simulink model "collagenSim"  (R2021b)
settings: Solver=VariableStepAuto  StartTime=0.0  StopTime=900  RelTol=1e-3
libraries: fl_lib x360, nesl_utility x174, rllib x1
(part 2 of 4)

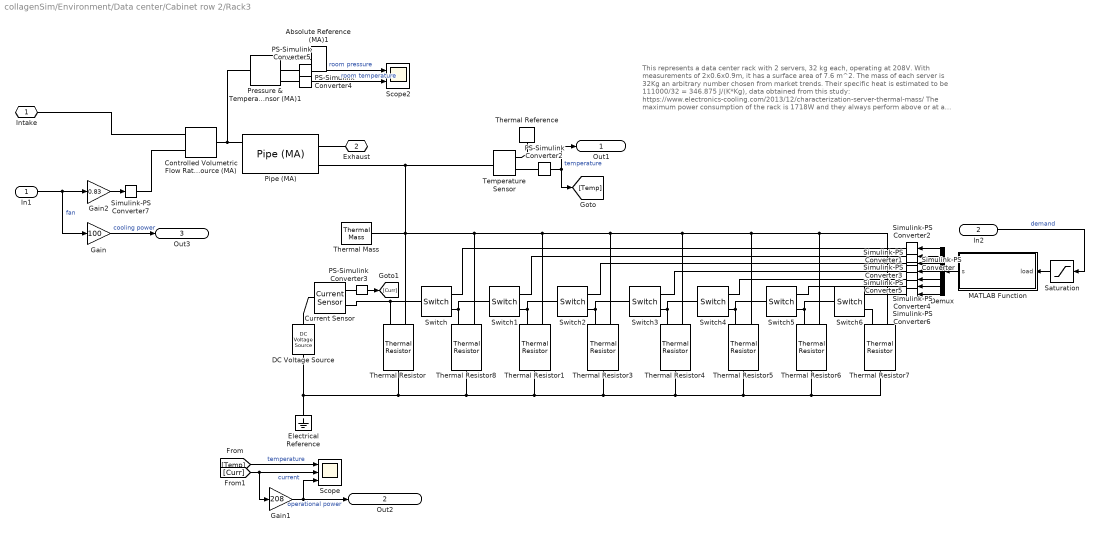
== system collagenSim/Environment/Data center/Cabinet row 2/Rack3 ==
  note: This represents a data center rack with 2 servers, 32 kg each, operating at 208V. With measurements of 2x0.6x0.9m, it has a surface area of 7.6 m^2. The mass of each server is 32Kg an arbitrary number chosen from market trends. Their specific heat is estimated to be 111000/32 = 346.875 J/(K*Kg), data obtained from this study: https://www.electronics-cooling.com/2013/12/characterization-server-thermal-mass/
      | The maximum power consumption of the rack is 1718W and they always perform above or at a minumum of 214.75W.
      | The rack's temperature exchange with the outside environment is modeled with a fluid pipe using the thermal propeties of air at sea level. The cooling system is modeled as eight 8mm four fan panels consuming a maximum of 100W per panel, which gives to each of the eight a total maximum vulumetric rate of 212m^3/min, meaning 0.83m^3/s. The surface area of the pipe representing the interior of the servers has been underestimated to be equal to the surface of the casing that contains them.
  In1 : Inport
  In2 : Inport  Port=2
  Absolute Reference (MA)1 : fl_lib/Moist Air/Elements/Absolute Reference (MA)
      settings: SourceProductBaseCode=SS
  Controlled Volumetric Flow Rate Source (MA) : fl_lib/Moist Air/Sources/Controlled Volumetric Flow Rate Source (MA)  power_spec=foundation.enum.power_spec.isentropic  volumetric_flow_conditions=foundation.enum.volumetric_flow_conditions.actual  p_std=0.101325 MPa  T_std=20 degC  RH_std=0.65  area_A=2*(2*0.442*0.4+2*0.442*0.711) m^2  area_B=2*(2*0.442*0.4+2*0.442*0.711) m^2
      settings: SourceProductBaseCode=SS  InternalSimscapePortConfiguration="{\"Bottom\":[],\"Left\":[{\"id\":\"A\",\"label\":\"A\",\"type\":\"foundation.moist_air.moist_air\"},{\"id\":\"V\",\"label\":\"V\",\"type\":\"input\"}],\"Right\":[{\"id\":\"B\",\"label\":\"B\",\"type\":\"foundation.moist_air.moist_air\"}],\"Top\":[]}"
  Current Sensor : fl_lib/Electrical/Electrical Sensors/Current Sensor
  DC Voltage Source : fl_lib/Electrical/Electrical Sources/DC Voltage Source  v0=208 V
  Demux : Demux  Outputs=7
  Electrical Reference : fl_lib/Electrical/Electrical Elements/Electrical Reference
  Gain : Gain  Gain=100
  Gain1 : Gain  Gain=208
  Gain2 : Gain  Gain=0.83
  MATLAB Function : MATLAB Function  TreatAsAtomicUnit=on
  PS-Simulink Converter{2..5} (4 alike) : nesl_utility/PS-Simulink Converter  PhysicalDomain=network_engine_domain  SubClassName=ps_output  LeftPortType=input  RightPortType=output  PseudoPeriodic=off  Frequencies=[]  Unit=inherit  AffineConversion=off
      settings: SourceProductBaseCode=PW,SS
  Pipe (MA) : fl_lib/Moist Air/Elements/Pipe (MA)  length=0.711 m  area=2*(2*0.442*0.4+2*0.442*0.711) m^2  Dh=0.1 m  length_add=0.1 m  roughness=15e-6 m  Re_lam=2000  Re_tur=4000  shape_factor=64  Nu_lam=3.66  RH_ws=1  time_constant=1e-3 s  moisture_trace_gas_source=foundation.enum.moisture_trace_gas_source.none  moisture_source_spec=foundation.enum.moisture_source_spec.vapor  moisture_mass_flow=0 kg/s  moisture_temperature_spec=foundation.enum.temperature_spec.atmospheric  moisture_temperature=293.15 K  trace_gas_mass_flow=0 kg/s  trace_gas_temperature_spec=foundation.enum.temperature_spec.atmospheric  trace_gas_temperature=293.15 K  p_I_specify=off  p_I_priority=High  p_I=0.101325 MPa  p_I_nominal_specify=off  p_I_nominal_unit=MPa  p_I_nominal_value=1  T_I_specify=off  T_I_priority=High  T_I=293.15 K  T_I_nominal_specify=off  T_I_nominal_unit=K  T_I_nominal_value=1  RH_I_specify=off  RH_I_priority=High  RH_I=0  RH_I_nominal_specify=off  RH_I_nominal_unit=1  RH_I_nominal_value=1  x_w_I_specify=off  x_w_I_priority=None  x_w_I=0  x_w_I_nominal_specify=off  x_w_I_nominal_unit=1  x_w_I_nominal_value=1  y_w_I_specify=off  y_w_I_priority=None  y_w_I=0  y_w_I_nominal_specify=off  y_w_I_nominal_unit=1  y_w_I_nominal_value=1  HR_I_specify=off  HR_I_priority=None  HR_I=0  HR_I_nominal_specify=off  HR_I_nominal_unit=1  HR_I_nominal_value=1  x_g_I_specify=off  x_g_I_priority=High  x_g_I=0  x_g_I_nominal_specify=off  x_g_I_nominal_unit=1  x_g_I_nominal_value=1  y_g_I_specify=off  y_g_I_priority=None  y_g_I=0  y_g_I_nominal_specify=off  y_g_I_nominal_unit=1  y_g_I_nominal_value=1
      settings: SourceProductBaseCode=SS
  Pressure & Temperature Sensor (MA)1 : fl_lib/Moist Air/Sensors/Pressure & Temperature Sensor (MA)
      settings: SourceProductBaseCode=SS  InternalSimscapePortConfiguration="{\"Bottom\":[],\"Left\":[{\"id\":\"A\",\"label\":\"A\",\"type\":\"foundation.moist_air.moist_air\"}],\"Right\":[{\"id\":\"B\",\"label\":\"B\",\"type\":\"foundation.moist_air.moist_air\"},{\"id\":\"P\",\"label\":\"P\",\"type\":\"output\"},{\"id\":\"T\",\"label\":\"T\",\"type\":\"output\"}],\"Top\":[]}"
  Saturation : Saturate  UpperLimit=0.99  LowerLimit=0.01
  Scope : Scope  NumInputPorts=3
  Scope2 : Scope  NumInputPorts=2
  Simulink-PS Converter{,1..7} (8 alike) : nesl_utility/Simulink-PS Converter  PhysicalDomain=network_engine_domain  SubClassName=ps_input  LeftPortType=input  RightPortType=output  PseudoPeriodic=off  Frequencies=[]  NoiseDistribution=none  NoiseParameters=[]  Unit=1  AffineConversion=off  FilteringAndDerivatives=provide  SimscapeFilterOrder=1  InputFilterTimeConstant=0.001  UdotUserProvided=0
      settings: SourceProductBaseCode=PW,SS
  Switch{,1..6} (7 alike) : fl_lib/Electrical/Electrical Elements/Switch  R_closed=0.01 Ohm  G_open=1e-8 1/Ohm  Threshold=0.5  i_specify=off  i_priority=None  i=0 A  i_nominal_specify=off  i_nominal_unit=A  i_nominal_value=1  v_specify=off  v_priority=None  v=0 V  v_nominal_specify=off  v_nominal_unit=V  v_nominal_value=1
  Temperature Sensor : fl_lib/Thermal/Thermal Sensors/Temperature Sensor
  Thermal Mass : fl_lib/Thermal/Thermal Elements/Thermal Mass  mass=64 kg  sp_heat=346.875 J/(K*kg)  T_specify=on  T_priority=High  T=293.15 K  T_nominal_specify=off  T_nominal_unit=K  T_nominal_value=1  Q_specify=off  Q_priority=None  Q=0 W  Q_nominal_specify=off  Q_nominal_unit=W  Q_nominal_value=1
  Thermal Reference : fl_lib/Thermal/Thermal Elements/Thermal Reference
  Thermal Resistor{,1,3..8} (8 alike) : fl_lib/Electrical/Electrical Elements/Thermal Resistor  R0=208^2/1718*8 Ohm  T0=298.15 K  alpha=50e-6 1/K  tc=10 s  K_d=1e-3 W/K  T_specify=on  T_priority=High  T=293.15 K  T_nominal_specify=off  T_nominal_unit=K  T_nominal_value=1
      settings: SourceProductBaseCode=SS  InternalSimscapePortConfiguration="{\"Bottom\":[],\"Left\":[{\"id\":\"H\",\"label\":\"H\",\"type\":\"foundation.thermal.thermal\"},{\"id\":\"p\",\"label\":\"+\",\"type\":\"foundation.electrical.electrical\"}],\"Right\":[{\"id\":\"n\",\"label\":\"-\",\"type\":\"foundation.electrical.electrical\"}],\"Top\":[]}"
  Intake : PMIOPort  Side=Left
  Exhaust : PMIOPort  Port=2  Side=Right
  Out1 : Outport
  Out2 : Outport  Port=2
  Out3 : Outport  Port=3
  wires:
  Demux/6 -> Simulink-PS Converter5/1
  Demux/1 -> Simulink-PS Converter2/1
  Demux/2 -> Simulink-PS Converter1/1
  Demux/7 -> Simulink-PS Converter6/1
  PS-Simulink Converter2/1 -> Out1/1, [Temp]  "temperature"
  [Curr] -> Scope/2, Gain1/1  "current"
  [Temp] -> Scope/1  "temperature"
  PS-Simulink Converter3/1 -> [Curr]
  Saturation/1 -> MATLAB Function/1(load)
  In2/1 -> Saturation/1  "demand"
  Demux/4 -> Simulink-PS Converter3/1
  Demux/3 -> Simulink-PS Converter/1
  Demux/5 -> Simulink-PS Converter4/1
  MATLAB Function/1(s) -> Demux/1
  Gain1/1 -> Out2/1, Scope/3  "operational power"
  In1/1 -> Gain/1, Gain2/1  "fan"
  Gain2/1 -> Simulink-PS Converter7/1
  Gain/1 -> Out3/1  "cooling power"
  PS-Simulink Converter5/1 -> Scope2/1  "room pressure"
  PS-Simulink Converter4/1 -> Scope2/2  "room temperature"
  connections:
  Switch3/LConn1 -- Switch2/RConn2 -- Thermal Resistor3/LConn2
  Thermal Resistor3/RConn1 -- Thermal Resistor6/RConn1 -- Thermal Resistor7/RConn1 -- Thermal Resistor5/RConn1 -- Thermal Resistor4/RConn1 -- Thermal Resistor8/RConn1 -- Electrical Reference/LConn1 -- DC Voltage Source/RConn1 -- Thermal Resistor/RConn1 -- Thermal Resistor1/RConn1
  DC Voltage Source/LConn1 -- Current Sensor/LConn1
  Switch2/LConn1 -- Switch1/RConn2 -- Thermal Resistor1/LConn2
  Switch1/LConn1 -- Switch/RConn2 -- Thermal Resistor8/LConn2
  Thermal Resistor4/LConn2 -- Switch4/LConn1 -- Switch3/RConn2
  Switch6/LConn1 -- Switch5/RConn2 -- Thermal Resistor6/LConn2
  Switch/LConn1 -- Current Sensor/RConn2 -- Thermal Resistor/LConn2
  Thermal Resistor5/LConn2 -- Switch5/LConn1 -- Switch4/RConn2
  Thermal Reference/LConn1 -- Temperature Sensor/RConn1
  Simulink-PS Converter6/RConn1 -- Switch6/RConn1
  Thermal Resistor7/LConn2 -- Switch6/RConn2
  Simulink-PS Converter4/RConn1 -- Switch4/RConn1
  Simulink-PS Converter2/RConn1 -- Switch/RConn1
  Simulink-PS Converter1/RConn1 -- Switch1/RConn1
  Temperature Sensor/RConn2 -- PS-Simulink Converter2/LConn1
  Simulink-PS Converter/RConn1 -- Switch2/RConn1
  Current Sensor/RConn1 -- PS-Simulink Converter3/LConn1
  Simulink-PS Converter3/RConn1 -- Switch3/RConn1
  Simulink-PS Converter5/RConn1 -- Switch5/RConn1
  Controlled Volumetric Flow Rate Source (MA)/LConn2 -- Simulink-PS Converter7/RConn1
  Pipe (MA)/RConn1 -- Controlled Volumetric Flow Rate Source (MA)/RConn1 -- Pressure & Temperature Sensor (MA)1/LConn1
  Intake/RConn1 -- Controlled Volumetric Flow Rate Source (MA)/LConn1
  Pipe (MA)/LConn1 -- Exhaust/RConn1
  Thermal Resistor8/LConn1 -- Pipe (MA)/LConn2 -- Temperature Sensor/LConn1 -- Thermal Resistor/LConn1 -- Thermal Mass/LConn1 -- Thermal Resistor6/LConn1 -- Thermal Resistor7/LConn1 -- Thermal Resistor5/LConn1 -- Thermal Resistor4/LConn1 -- Thermal Resistor3/LConn1 -- Thermal Resistor1/LConn1
  PS-Simulink Converter5/LConn1 -- Pressure & Temperature Sensor (MA)1/RConn2
  PS-Simulink Converter4/LConn1 -- Pressure & Temperature Sensor (MA)1/RConn3
  Absolute Reference (MA)1/LConn1 -- Pressure & Temperature Sensor (MA)1/RConn1

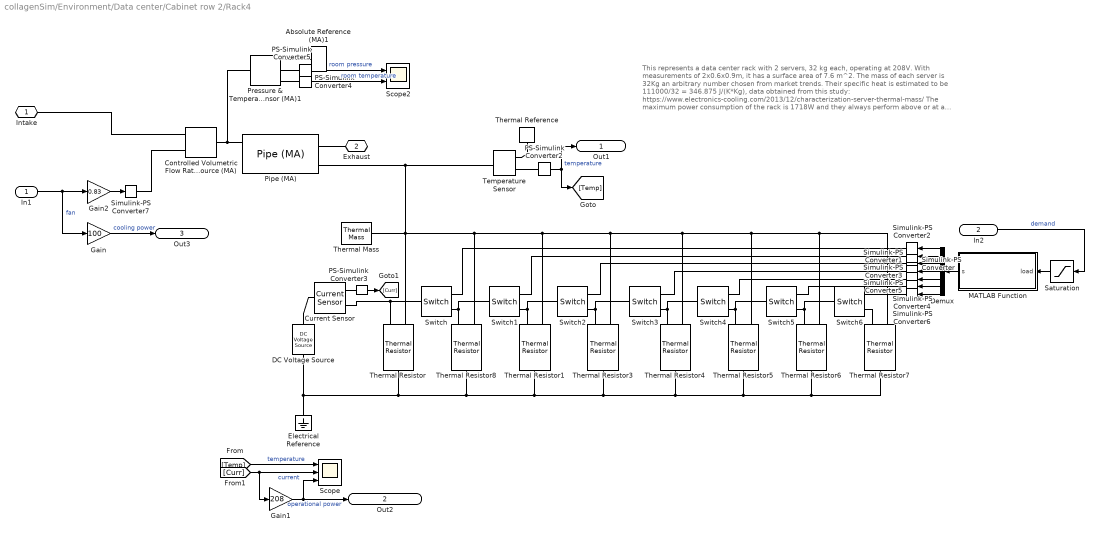
== system collagenSim/Environment/Data center/Cabinet row 2/Rack4 ==
  note: This represents a data center rack with 2 servers, 32 kg each, operating at 208V. With measurements of 2x0.6x0.9m, it has a surface area of 7.6 m^2. The mass of each server is 32Kg an arbitrary number chosen from market trends. Their specific heat is estimated to be 111000/32 = 346.875 J/(K*Kg), data obtained from this study: https://www.electronics-cooling.com/2013/12/characterization-server-thermal-mass/
      | The maximum power consumption of the rack is 1718W and they always perform above or at a minumum of 214.75W.
      | The rack's temperature exchange with the outside environment is modeled with a fluid pipe using the thermal propeties of air at sea level. The cooling system is modeled as eight 8mm four fan panels consuming a maximum of 100W per panel, which gives to each of the eight a total maximum vulumetric rate of 212m^3/min, meaning 0.83m^3/s. The surface area of the pipe representing the interior of the servers has been underestimated to be equal to the surface of the casing that contains them.
  In1 : Inport
  In2 : Inport  Port=2
  Absolute Reference (MA)1 : fl_lib/Moist Air/Elements/Absolute Reference (MA)
      settings: SourceProductBaseCode=SS
  Controlled Volumetric Flow Rate Source (MA) : fl_lib/Moist Air/Sources/Controlled Volumetric Flow Rate Source (MA)  power_spec=foundation.enum.power_spec.isentropic  volumetric_flow_conditions=foundation.enum.volumetric_flow_conditions.actual  p_std=0.101325 MPa  T_std=20 degC  RH_std=0.65  area_A=2*(2*0.442*0.4+2*0.442*0.711) m^2  area_B=2*(2*0.442*0.4+2*0.442*0.711) m^2
      settings: SourceProductBaseCode=SS  InternalSimscapePortConfiguration="{\"Bottom\":[],\"Left\":[{\"id\":\"A\",\"label\":\"A\",\"type\":\"foundation.moist_air.moist_air\"},{\"id\":\"V\",\"label\":\"V\",\"type\":\"input\"}],\"Right\":[{\"id\":\"B\",\"label\":\"B\",\"type\":\"foundation.moist_air.moist_air\"}],\"Top\":[]}"
  Current Sensor : fl_lib/Electrical/Electrical Sensors/Current Sensor
  DC Voltage Source : fl_lib/Electrical/Electrical Sources/DC Voltage Source  v0=208 V
  Demux : Demux  Outputs=7
  Electrical Reference : fl_lib/Electrical/Electrical Elements/Electrical Reference
  Gain : Gain  Gain=100
  Gain1 : Gain  Gain=208
  Gain2 : Gain  Gain=0.83
  MATLAB Function : MATLAB Function  TreatAsAtomicUnit=on
  PS-Simulink Converter{2..5} (4 alike) : nesl_utility/PS-Simulink Converter  PhysicalDomain=network_engine_domain  SubClassName=ps_output  LeftPortType=input  RightPortType=output  PseudoPeriodic=off  Frequencies=[]  Unit=inherit  AffineConversion=off
      settings: SourceProductBaseCode=PW,SS
  Pipe (MA) : fl_lib/Moist Air/Elements/Pipe (MA)  length=0.711 m  area=2*(2*0.442*0.4+2*0.442*0.711) m^2  Dh=0.1 m  length_add=0.1 m  roughness=15e-6 m  Re_lam=2000  Re_tur=4000  shape_factor=64  Nu_lam=3.66  RH_ws=1  time_constant=1e-3 s  moisture_trace_gas_source=foundation.enum.moisture_trace_gas_source.none  moisture_source_spec=foundation.enum.moisture_source_spec.vapor  moisture_mass_flow=0 kg/s  moisture_temperature_spec=foundation.enum.temperature_spec.atmospheric  moisture_temperature=293.15 K  trace_gas_mass_flow=0 kg/s  trace_gas_temperature_spec=foundation.enum.temperature_spec.atmospheric  trace_gas_temperature=293.15 K  p_I_specify=off  p_I_priority=High  p_I=0.101325 MPa  p_I_nominal_specify=off  p_I_nominal_unit=MPa  p_I_nominal_value=1  T_I_specify=off  T_I_priority=High  T_I=293.15 K  T_I_nominal_specify=off  T_I_nominal_unit=K  T_I_nominal_value=1  RH_I_specify=off  RH_I_priority=High  RH_I=0  RH_I_nominal_specify=off  RH_I_nominal_unit=1  RH_I_nominal_value=1  x_w_I_specify=off  x_w_I_priority=None  x_w_I=0  x_w_I_nominal_specify=off  x_w_I_nominal_unit=1  x_w_I_nominal_value=1  y_w_I_specify=off  y_w_I_priority=None  y_w_I=0  y_w_I_nominal_specify=off  y_w_I_nominal_unit=1  y_w_I_nominal_value=1  HR_I_specify=off  HR_I_priority=None  HR_I=0  HR_I_nominal_specify=off  HR_I_nominal_unit=1  HR_I_nominal_value=1  x_g_I_specify=off  x_g_I_priority=High  x_g_I=0  x_g_I_nominal_specify=off  x_g_I_nominal_unit=1  x_g_I_nominal_value=1  y_g_I_specify=off  y_g_I_priority=None  y_g_I=0  y_g_I_nominal_specify=off  y_g_I_nominal_unit=1  y_g_I_nominal_value=1
      settings: SourceProductBaseCode=SS
  Pressure & Temperature Sensor (MA)1 : fl_lib/Moist Air/Sensors/Pressure & Temperature Sensor (MA)
      settings: SourceProductBaseCode=SS  InternalSimscapePortConfiguration="{\"Bottom\":[],\"Left\":[{\"id\":\"A\",\"label\":\"A\",\"type\":\"foundation.moist_air.moist_air\"}],\"Right\":[{\"id\":\"B\",\"label\":\"B\",\"type\":\"foundation.moist_air.moist_air\"},{\"id\":\"P\",\"label\":\"P\",\"type\":\"output\"},{\"id\":\"T\",\"label\":\"T\",\"type\":\"output\"}],\"Top\":[]}"
  Saturation : Saturate  UpperLimit=0.99  LowerLimit=0.01
  Scope : Scope  NumInputPorts=3
  Scope2 : Scope  NumInputPorts=2
  Simulink-PS Converter{,1..7} (8 alike) : nesl_utility/Simulink-PS Converter  PhysicalDomain=network_engine_domain  SubClassName=ps_input  LeftPortType=input  RightPortType=output  PseudoPeriodic=off  Frequencies=[]  NoiseDistribution=none  NoiseParameters=[]  Unit=1  AffineConversion=off  FilteringAndDerivatives=provide  SimscapeFilterOrder=1  InputFilterTimeConstant=0.001  UdotUserProvided=0
      settings: SourceProductBaseCode=PW,SS
  Switch{,1..6} (7 alike) : fl_lib/Electrical/Electrical Elements/Switch  R_closed=0.01 Ohm  G_open=1e-8 1/Ohm  Threshold=0.5  i_specify=off  i_priority=None  i=0 A  i_nominal_specify=off  i_nominal_unit=A  i_nominal_value=1  v_specify=off  v_priority=None  v=0 V  v_nominal_specify=off  v_nominal_unit=V  v_nominal_value=1
  Temperature Sensor : fl_lib/Thermal/Thermal Sensors/Temperature Sensor
  Thermal Mass : fl_lib/Thermal/Thermal Elements/Thermal Mass  mass=64 kg  sp_heat=346.875 J/(K*kg)  T_specify=on  T_priority=High  T=293.15 K  T_nominal_specify=off  T_nominal_unit=K  T_nominal_value=1  Q_specify=off  Q_priority=None  Q=0 W  Q_nominal_specify=off  Q_nominal_unit=W  Q_nominal_value=1
  Thermal Reference : fl_lib/Thermal/Thermal Elements/Thermal Reference
  Thermal Resistor{,1,3..8} (8 alike) : fl_lib/Electrical/Electrical Elements/Thermal Resistor  R0=208^2/1718*8 Ohm  T0=298.15 K  alpha=50e-6 1/K  tc=10 s  K_d=1e-3 W/K  T_specify=on  T_priority=High  T=293.15 K  T_nominal_specify=off  T_nominal_unit=K  T_nominal_value=1
      settings: SourceProductBaseCode=SS  InternalSimscapePortConfiguration="{\"Bottom\":[],\"Left\":[{\"id\":\"H\",\"label\":\"H\",\"type\":\"foundation.thermal.thermal\"},{\"id\":\"p\",\"label\":\"+\",\"type\":\"foundation.electrical.electrical\"}],\"Right\":[{\"id\":\"n\",\"label\":\"-\",\"type\":\"foundation.electrical.electrical\"}],\"Top\":[]}"
  Intake : PMIOPort  Side=Left
  Exhaust : PMIOPort  Port=2  Side=Right
  Out1 : Outport
  Out2 : Outport  Port=2
  Out3 : Outport  Port=3
  wires:
  Demux/6 -> Simulink-PS Converter5/1
  Demux/1 -> Simulink-PS Converter2/1
  Demux/2 -> Simulink-PS Converter1/1
  Demux/7 -> Simulink-PS Converter6/1
  PS-Simulink Converter2/1 -> Out1/1, [Temp]  "temperature"
  [Curr] -> Scope/2, Gain1/1  "current"
  [Temp] -> Scope/1  "temperature"
  PS-Simulink Converter3/1 -> [Curr]
  Saturation/1 -> MATLAB Function/1(load)
  In2/1 -> Saturation/1  "demand"
  Demux/4 -> Simulink-PS Converter3/1
  Demux/3 -> Simulink-PS Converter/1
  Demux/5 -> Simulink-PS Converter4/1
  MATLAB Function/1(s) -> Demux/1
  Gain1/1 -> Out2/1, Scope/3  "operational power"
  In1/1 -> Gain/1, Gain2/1  "fan"
  Gain2/1 -> Simulink-PS Converter7/1
  Gain/1 -> Out3/1  "cooling power"
  PS-Simulink Converter5/1 -> Scope2/1  "room pressure"
  PS-Simulink Converter4/1 -> Scope2/2  "room temperature"
  connections:
  Switch3/LConn1 -- Switch2/RConn2 -- Thermal Resistor3/LConn2
  Thermal Resistor3/RConn1 -- Thermal Resistor6/RConn1 -- Thermal Resistor7/RConn1 -- Thermal Resistor5/RConn1 -- Thermal Resistor4/RConn1 -- Thermal Resistor8/RConn1 -- Electrical Reference/LConn1 -- DC Voltage Source/RConn1 -- Thermal Resistor/RConn1 -- Thermal Resistor1/RConn1
  DC Voltage Source/LConn1 -- Current Sensor/LConn1
  Switch2/LConn1 -- Switch1/RConn2 -- Thermal Resistor1/LConn2
  Switch1/LConn1 -- Switch/RConn2 -- Thermal Resistor8/LConn2
  Thermal Resistor4/LConn2 -- Switch4/LConn1 -- Switch3/RConn2
  Switch6/LConn1 -- Switch5/RConn2 -- Thermal Resistor6/LConn2
  Switch/LConn1 -- Current Sensor/RConn2 -- Thermal Resistor/LConn2
  Thermal Resistor5/LConn2 -- Switch5/LConn1 -- Switch4/RConn2
  Thermal Reference/LConn1 -- Temperature Sensor/RConn1
  Simulink-PS Converter6/RConn1 -- Switch6/RConn1
  Thermal Resistor7/LConn2 -- Switch6/RConn2
  Simulink-PS Converter4/RConn1 -- Switch4/RConn1
  Simulink-PS Converter2/RConn1 -- Switch/RConn1
  Simulink-PS Converter1/RConn1 -- Switch1/RConn1
  Temperature Sensor/RConn2 -- PS-Simulink Converter2/LConn1
  Simulink-PS Converter/RConn1 -- Switch2/RConn1
  Current Sensor/RConn1 -- PS-Simulink Converter3/LConn1
  Simulink-PS Converter3/RConn1 -- Switch3/RConn1
  Simulink-PS Converter5/RConn1 -- Switch5/RConn1
  Controlled Volumetric Flow Rate Source (MA)/LConn2 -- Simulink-PS Converter7/RConn1
  Pipe (MA)/RConn1 -- Controlled Volumetric Flow Rate Source (MA)/RConn1 -- Pressure & Temperature Sensor (MA)1/LConn1
  Intake/RConn1 -- Controlled Volumetric Flow Rate Source (MA)/LConn1
  Pipe (MA)/LConn1 -- Exhaust/RConn1
  Thermal Resistor8/LConn1 -- Pipe (MA)/LConn2 -- Temperature Sensor/LConn1 -- Thermal Resistor/LConn1 -- Thermal Mass/LConn1 -- Thermal Resistor6/LConn1 -- Thermal Resistor7/LConn1 -- Thermal Resistor5/LConn1 -- Thermal Resistor4/LConn1 -- Thermal Resistor3/LConn1 -- Thermal Resistor1/LConn1
  PS-Simulink Converter5/LConn1 -- Pressure & Temperature Sensor (MA)1/RConn2
  PS-Simulink Converter4/LConn1 -- Pressure & Temperature Sensor (MA)1/RConn3
  Absolute Reference (MA)1/LConn1 -- Pressure & Temperature Sensor (MA)1/RConn1

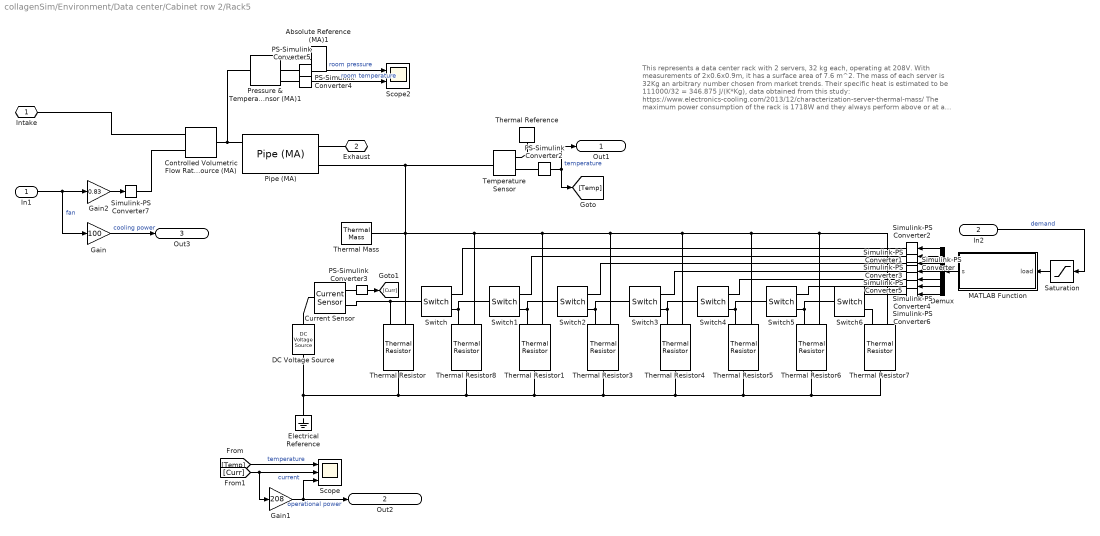
== system collagenSim/Environment/Data center/Cabinet row 2/Rack5 ==
  note: This represents a data center rack with 2 servers, 32 kg each, operating at 208V. With measurements of 2x0.6x0.9m, it has a surface area of 7.6 m^2. The mass of each server is 32Kg an arbitrary number chosen from market trends. Their specific heat is estimated to be 111000/32 = 346.875 J/(K*Kg), data obtained from this study: https://www.electronics-cooling.com/2013/12/characterization-server-thermal-mass/
      | The maximum power consumption of the rack is 1718W and they always perform above or at a minumum of 214.75W.
      | The rack's temperature exchange with the outside environment is modeled with a fluid pipe using the thermal propeties of air at sea level. The cooling system is modeled as eight 8mm four fan panels consuming a maximum of 100W per panel, which gives to each of the eight a total maximum vulumetric rate of 212m^3/min, meaning 0.83m^3/s. The surface area of the pipe representing the interior of the servers has been underestimated to be equal to the surface of the casing that contains them.
  In1 : Inport
  In2 : Inport  Port=2
  Absolute Reference (MA)1 : fl_lib/Moist Air/Elements/Absolute Reference (MA)
      settings: SourceProductBaseCode=SS
  Controlled Volumetric Flow Rate Source (MA) : fl_lib/Moist Air/Sources/Controlled Volumetric Flow Rate Source (MA)  power_spec=foundation.enum.power_spec.isentropic  volumetric_flow_conditions=foundation.enum.volumetric_flow_conditions.actual  p_std=0.101325 MPa  T_std=20 degC  RH_std=0.65  area_A=2*(2*0.442*0.4+2*0.442*0.711) m^2  area_B=2*(2*0.442*0.4+2*0.442*0.711) m^2
      settings: SourceProductBaseCode=SS  InternalSimscapePortConfiguration="{\"Bottom\":[],\"Left\":[{\"id\":\"A\",\"label\":\"A\",\"type\":\"foundation.moist_air.moist_air\"},{\"id\":\"V\",\"label\":\"V\",\"type\":\"input\"}],\"Right\":[{\"id\":\"B\",\"label\":\"B\",\"type\":\"foundation.moist_air.moist_air\"}],\"Top\":[]}"
  Current Sensor : fl_lib/Electrical/Electrical Sensors/Current Sensor
  DC Voltage Source : fl_lib/Electrical/Electrical Sources/DC Voltage Source  v0=208 V
  Demux : Demux  Outputs=7
  Electrical Reference : fl_lib/Electrical/Electrical Elements/Electrical Reference
  Gain : Gain  Gain=100
  Gain1 : Gain  Gain=208
  Gain2 : Gain  Gain=0.83
  MATLAB Function : MATLAB Function  TreatAsAtomicUnit=on
  PS-Simulink Converter{2..5} (4 alike) : nesl_utility/PS-Simulink Converter  PhysicalDomain=network_engine_domain  SubClassName=ps_output  LeftPortType=input  RightPortType=output  PseudoPeriodic=off  Frequencies=[]  Unit=inherit  AffineConversion=off
      settings: SourceProductBaseCode=PW,SS
  Pipe (MA) : fl_lib/Moist Air/Elements/Pipe (MA)  length=0.711 m  area=2*(2*0.442*0.4+2*0.442*0.711) m^2  Dh=0.1 m  length_add=0.1 m  roughness=15e-6 m  Re_lam=2000  Re_tur=4000  shape_factor=64  Nu_lam=3.66  RH_ws=1  time_constant=1e-3 s  moisture_trace_gas_source=foundation.enum.moisture_trace_gas_source.none  moisture_source_spec=foundation.enum.moisture_source_spec.vapor  moisture_mass_flow=0 kg/s  moisture_temperature_spec=foundation.enum.temperature_spec.atmospheric  moisture_temperature=293.15 K  trace_gas_mass_flow=0 kg/s  trace_gas_temperature_spec=foundation.enum.temperature_spec.atmospheric  trace_gas_temperature=293.15 K  p_I_specify=off  p_I_priority=High  p_I=0.101325 MPa  p_I_nominal_specify=off  p_I_nominal_unit=MPa  p_I_nominal_value=1  T_I_specify=off  T_I_priority=High  T_I=293.15 K  T_I_nominal_specify=off  T_I_nominal_unit=K  T_I_nominal_value=1  RH_I_specify=off  RH_I_priority=High  RH_I=0  RH_I_nominal_specify=off  RH_I_nominal_unit=1  RH_I_nominal_value=1  x_w_I_specify=off  x_w_I_priority=None  x_w_I=0  x_w_I_nominal_specify=off  x_w_I_nominal_unit=1  x_w_I_nominal_value=1  y_w_I_specify=off  y_w_I_priority=None  y_w_I=0  y_w_I_nominal_specify=off  y_w_I_nominal_unit=1  y_w_I_nominal_value=1  HR_I_specify=off  HR_I_priority=None  HR_I=0  HR_I_nominal_specify=off  HR_I_nominal_unit=1  HR_I_nominal_value=1  x_g_I_specify=off  x_g_I_priority=High  x_g_I=0  x_g_I_nominal_specify=off  x_g_I_nominal_unit=1  x_g_I_nominal_value=1  y_g_I_specify=off  y_g_I_priority=None  y_g_I=0  y_g_I_nominal_specify=off  y_g_I_nominal_unit=1  y_g_I_nominal_value=1
      settings: SourceProductBaseCode=SS
  Pressure & Temperature Sensor (MA)1 : fl_lib/Moist Air/Sensors/Pressure & Temperature Sensor (MA)
      settings: SourceProductBaseCode=SS  InternalSimscapePortConfiguration="{\"Bottom\":[],\"Left\":[{\"id\":\"A\",\"label\":\"A\",\"type\":\"foundation.moist_air.moist_air\"}],\"Right\":[{\"id\":\"B\",\"label\":\"B\",\"type\":\"foundation.moist_air.moist_air\"},{\"id\":\"P\",\"label\":\"P\",\"type\":\"output\"},{\"id\":\"T\",\"label\":\"T\",\"type\":\"output\"}],\"Top\":[]}"
  Saturation : Saturate  UpperLimit=0.99  LowerLimit=0.01
  Scope : Scope  NumInputPorts=3
  Scope2 : Scope  NumInputPorts=2
  Simulink-PS Converter{,1..7} (8 alike) : nesl_utility/Simulink-PS Converter  PhysicalDomain=network_engine_domain  SubClassName=ps_input  LeftPortType=input  RightPortType=output  PseudoPeriodic=off  Frequencies=[]  NoiseDistribution=none  NoiseParameters=[]  Unit=1  AffineConversion=off  FilteringAndDerivatives=provide  SimscapeFilterOrder=1  InputFilterTimeConstant=0.001  UdotUserProvided=0
      settings: SourceProductBaseCode=PW,SS
  Switch{,1..6} (7 alike) : fl_lib/Electrical/Electrical Elements/Switch  R_closed=0.01 Ohm  G_open=1e-8 1/Ohm  Threshold=0.5  i_specify=off  i_priority=None  i=0 A  i_nominal_specify=off  i_nominal_unit=A  i_nominal_value=1  v_specify=off  v_priority=None  v=0 V  v_nominal_specify=off  v_nominal_unit=V  v_nominal_value=1
  Temperature Sensor : fl_lib/Thermal/Thermal Sensors/Temperature Sensor
  Thermal Mass : fl_lib/Thermal/Thermal Elements/Thermal Mass  mass=64 kg  sp_heat=346.875 J/(K*kg)  T_specify=on  T_priority=High  T=293.15 K  T_nominal_specify=off  T_nominal_unit=K  T_nominal_value=1  Q_specify=off  Q_priority=None  Q=0 W  Q_nominal_specify=off  Q_nominal_unit=W  Q_nominal_value=1
  Thermal Reference : fl_lib/Thermal/Thermal Elements/Thermal Reference
  Thermal Resistor{,1,3..8} (8 alike) : fl_lib/Electrical/Electrical Elements/Thermal Resistor  R0=208^2/1718*8 Ohm  T0=298.15 K  alpha=50e-6 1/K  tc=10 s  K_d=1e-3 W/K  T_specify=on  T_priority=High  T=293.15 K  T_nominal_specify=off  T_nominal_unit=K  T_nominal_value=1
      settings: SourceProductBaseCode=SS  InternalSimscapePortConfiguration="{\"Bottom\":[],\"Left\":[{\"id\":\"H\",\"label\":\"H\",\"type\":\"foundation.thermal.thermal\"},{\"id\":\"p\",\"label\":\"+\",\"type\":\"foundation.electrical.electrical\"}],\"Right\":[{\"id\":\"n\",\"label\":\"-\",\"type\":\"foundation.electrical.electrical\"}],\"Top\":[]}"
  Intake : PMIOPort  Side=Left
  Exhaust : PMIOPort  Port=2  Side=Right
  Out1 : Outport
  Out2 : Outport  Port=2
  Out3 : Outport  Port=3
  wires:
  Demux/6 -> Simulink-PS Converter5/1
  Demux/1 -> Simulink-PS Converter2/1
  Demux/2 -> Simulink-PS Converter1/1
  Demux/7 -> Simulink-PS Converter6/1
  PS-Simulink Converter2/1 -> Out1/1, [Temp]  "temperature"
  [Curr] -> Scope/2, Gain1/1  "current"
  [Temp] -> Scope/1  "temperature"
  PS-Simulink Converter3/1 -> [Curr]
  Saturation/1 -> MATLAB Function/1(load)
  In2/1 -> Saturation/1  "demand"
  Demux/4 -> Simulink-PS Converter3/1
  Demux/3 -> Simulink-PS Converter/1
  Demux/5 -> Simulink-PS Converter4/1
  MATLAB Function/1(s) -> Demux/1
  Gain1/1 -> Out2/1, Scope/3  "operational power"
  In1/1 -> Gain/1, Gain2/1  "fan"
  Gain2/1 -> Simulink-PS Converter7/1
  Gain/1 -> Out3/1  "cooling power"
  PS-Simulink Converter5/1 -> Scope2/1  "room pressure"
  PS-Simulink Converter4/1 -> Scope2/2  "room temperature"
  connections:
  Switch3/LConn1 -- Switch2/RConn2 -- Thermal Resistor3/LConn2
  Thermal Resistor3/RConn1 -- Thermal Resistor6/RConn1 -- Thermal Resistor7/RConn1 -- Thermal Resistor5/RConn1 -- Thermal Resistor4/RConn1 -- Thermal Resistor8/RConn1 -- Electrical Reference/LConn1 -- DC Voltage Source/RConn1 -- Thermal Resistor/RConn1 -- Thermal Resistor1/RConn1
  DC Voltage Source/LConn1 -- Current Sensor/LConn1
  Switch2/LConn1 -- Switch1/RConn2 -- Thermal Resistor1/LConn2
  Switch1/LConn1 -- Switch/RConn2 -- Thermal Resistor8/LConn2
  Thermal Resistor4/LConn2 -- Switch4/LConn1 -- Switch3/RConn2
  Switch6/LConn1 -- Switch5/RConn2 -- Thermal Resistor6/LConn2
  Switch/LConn1 -- Current Sensor/RConn2 -- Thermal Resistor/LConn2
  Thermal Resistor5/LConn2 -- Switch5/LConn1 -- Switch4/RConn2
  Thermal Reference/LConn1 -- Temperature Sensor/RConn1
  Simulink-PS Converter6/RConn1 -- Switch6/RConn1
  Thermal Resistor7/LConn2 -- Switch6/RConn2
  Simulink-PS Converter4/RConn1 -- Switch4/RConn1
  Simulink-PS Converter2/RConn1 -- Switch/RConn1
  Simulink-PS Converter1/RConn1 -- Switch1/RConn1
  Temperature Sensor/RConn2 -- PS-Simulink Converter2/LConn1
  Simulink-PS Converter/RConn1 -- Switch2/RConn1
  Current Sensor/RConn1 -- PS-Simulink Converter3/LConn1
  Simulink-PS Converter3/RConn1 -- Switch3/RConn1
  Simulink-PS Converter5/RConn1 -- Switch5/RConn1
  Controlled Volumetric Flow Rate Source (MA)/LConn2 -- Simulink-PS Converter7/RConn1
  Pipe (MA)/RConn1 -- Controlled Volumetric Flow Rate Source (MA)/RConn1 -- Pressure & Temperature Sensor (MA)1/LConn1
  Intake/RConn1 -- Controlled Volumetric Flow Rate Source (MA)/LConn1
  Pipe (MA)/LConn1 -- Exhaust/RConn1
  Thermal Resistor8/LConn1 -- Pipe (MA)/LConn2 -- Temperature Sensor/LConn1 -- Thermal Resistor/LConn1 -- Thermal Mass/LConn1 -- Thermal Resistor6/LConn1 -- Thermal Resistor7/LConn1 -- Thermal Resistor5/LConn1 -- Thermal Resistor4/LConn1 -- Thermal Resistor3/LConn1 -- Thermal Resistor1/LConn1
  PS-Simulink Converter5/LConn1 -- Pressure & Temperature Sensor (MA)1/RConn2
  PS-Simulink Converter4/LConn1 -- Pressure & Temperature Sensor (MA)1/RConn3
  Absolute Reference (MA)1/LConn1 -- Pressure & Temperature Sensor (MA)1/RConn1

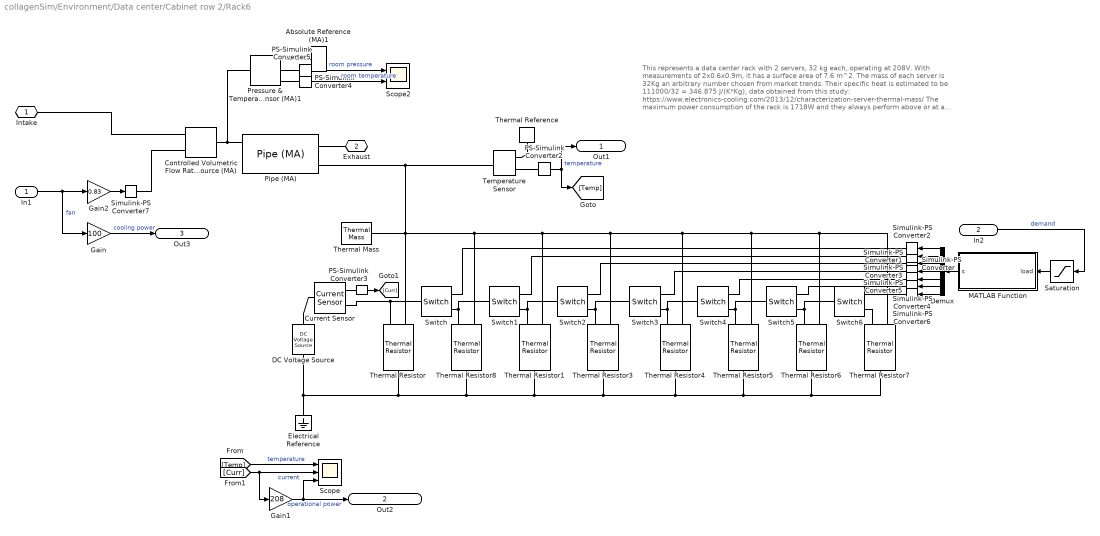
== system collagenSim/Environment/Data center/Cabinet row 2/Rack6 ==
  note: This represents a data center rack with 2 servers, 32 kg each, operating at 208V. With measurements of 2x0.6x0.9m, it has a surface area of 7.6 m^2. The mass of each server is 32Kg an arbitrary number chosen from market trends. Their specific heat is estimated to be 111000/32 = 346.875 J/(K*Kg), data obtained from this study: https://www.electronics-cooling.com/2013/12/characterization-server-thermal-mass/
      | The maximum power consumption of the rack is 1718W and they always perform above or at a minumum of 214.75W.
      | The rack's temperature exchange with the outside environment is modeled with a fluid pipe using the thermal propeties of air at sea level. The cooling system is modeled as eight 8mm four fan panels consuming a maximum of 100W per panel, which gives to each of the eight a total maximum vulumetric rate of 212m^3/min, meaning 0.83m^3/s. The surface area of the pipe representing the interior of the servers has been underestimated to be equal to the surface of the casing that contains them.
  In1 : Inport
  In2 : Inport  Port=2
  Absolute Reference (MA)1 : fl_lib/Moist Air/Elements/Absolute Reference (MA)
      settings: SourceProductBaseCode=SS
  Controlled Volumetric Flow Rate Source (MA) : fl_lib/Moist Air/Sources/Controlled Volumetric Flow Rate Source (MA)  power_spec=foundation.enum.power_spec.isentropic  volumetric_flow_conditions=foundation.enum.volumetric_flow_conditions.actual  p_std=0.101325 MPa  T_std=20 degC  RH_std=0.65  area_A=2*(2*0.442*0.4+2*0.442*0.711) m^2  area_B=2*(2*0.442*0.4+2*0.442*0.711) m^2
      settings: SourceProductBaseCode=SS  InternalSimscapePortConfiguration="{\"Bottom\":[],\"Left\":[{\"id\":\"A\",\"label\":\"A\",\"type\":\"foundation.moist_air.moist_air\"},{\"id\":\"V\",\"label\":\"V\",\"type\":\"input\"}],\"Right\":[{\"id\":\"B\",\"label\":\"B\",\"type\":\"foundation.moist_air.moist_air\"}],\"Top\":[]}"
  Current Sensor : fl_lib/Electrical/Electrical Sensors/Current Sensor
  DC Voltage Source : fl_lib/Electrical/Electrical Sources/DC Voltage Source  v0=208 V
  Demux : Demux  Outputs=7
  Electrical Reference : fl_lib/Electrical/Electrical Elements/Electrical Reference
  Gain : Gain  Gain=100
  Gain1 : Gain  Gain=208
  Gain2 : Gain  Gain=0.83
  MATLAB Function : MATLAB Function  TreatAsAtomicUnit=on
  PS-Simulink Converter{2..5} (4 alike) : nesl_utility/PS-Simulink Converter  PhysicalDomain=network_engine_domain  SubClassName=ps_output  LeftPortType=input  RightPortType=output  PseudoPeriodic=off  Frequencies=[]  Unit=inherit  AffineConversion=off
      settings: SourceProductBaseCode=PW,SS
  Pipe (MA) : fl_lib/Moist Air/Elements/Pipe (MA)  length=0.711 m  area=2*(2*0.442*0.4+2*0.442*0.711) m^2  Dh=0.1 m  length_add=0.1 m  roughness=15e-6 m  Re_lam=2000  Re_tur=4000  shape_factor=64  Nu_lam=3.66  RH_ws=1  time_constant=1e-3 s  moisture_trace_gas_source=foundation.enum.moisture_trace_gas_source.none  moisture_source_spec=foundation.enum.moisture_source_spec.vapor  moisture_mass_flow=0 kg/s  moisture_temperature_spec=foundation.enum.temperature_spec.atmospheric  moisture_temperature=293.15 K  trace_gas_mass_flow=0 kg/s  trace_gas_temperature_spec=foundation.enum.temperature_spec.atmospheric  trace_gas_temperature=293.15 K  p_I_specify=off  p_I_priority=High  p_I=0.101325 MPa  p_I_nominal_specify=off  p_I_nominal_unit=MPa  p_I_nominal_value=1  T_I_specify=off  T_I_priority=High  T_I=293.15 K  T_I_nominal_specify=off  T_I_nominal_unit=K  T_I_nominal_value=1  RH_I_specify=off  RH_I_priority=High  RH_I=0  RH_I_nominal_specify=off  RH_I_nominal_unit=1  RH_I_nominal_value=1  x_w_I_specify=off  x_w_I_priority=None  x_w_I=0  x_w_I_nominal_specify=off  x_w_I_nominal_unit=1  x_w_I_nominal_value=1  y_w_I_specify=off  y_w_I_priority=None  y_w_I=0  y_w_I_nominal_specify=off  y_w_I_nominal_unit=1  y_w_I_nominal_value=1  HR_I_specify=off  HR_I_priority=None  HR_I=0  HR_I_nominal_specify=off  HR_I_nominal_unit=1  HR_I_nominal_value=1  x_g_I_specify=off  x_g_I_priority=High  x_g_I=0  x_g_I_nominal_specify=off  x_g_I_nominal_unit=1  x_g_I_nominal_value=1  y_g_I_specify=off  y_g_I_priority=None  y_g_I=0  y_g_I_nominal_specify=off  y_g_I_nominal_unit=1  y_g_I_nominal_value=1
      settings: SourceProductBaseCode=SS
  Pressure & Temperature Sensor (MA)1 : fl_lib/Moist Air/Sensors/Pressure & Temperature Sensor (MA)
      settings: SourceProductBaseCode=SS  InternalSimscapePortConfiguration="{\"Bottom\":[],\"Left\":[{\"id\":\"A\",\"label\":\"A\",\"type\":\"foundation.moist_air.moist_air\"}],\"Right\":[{\"id\":\"B\",\"label\":\"B\",\"type\":\"foundation.moist_air.moist_air\"},{\"id\":\"P\",\"label\":\"P\",\"type\":\"output\"},{\"id\":\"T\",\"label\":\"T\",\"type\":\"output\"}],\"Top\":[]}"
  Saturation : Saturate  UpperLimit=0.99  LowerLimit=0.01
  Scope : Scope  NumInputPorts=3
  Scope2 : Scope  NumInputPorts=2
  Simulink-PS Converter{,1..7} (8 alike) : nesl_utility/Simulink-PS Converter  PhysicalDomain=network_engine_domain  SubClassName=ps_input  LeftPortType=input  RightPortType=output  PseudoPeriodic=off  Frequencies=[]  NoiseDistribution=none  NoiseParameters=[]  Unit=1  AffineConversion=off  FilteringAndDerivatives=provide  SimscapeFilterOrder=1  InputFilterTimeConstant=0.001  UdotUserProvided=0
      settings: SourceProductBaseCode=PW,SS
  Switch{,1..6} (7 alike) : fl_lib/Electrical/Electrical Elements/Switch  R_closed=0.01 Ohm  G_open=1e-8 1/Ohm  Threshold=0.5  i_specify=off  i_priority=None  i=0 A  i_nominal_specify=off  i_nominal_unit=A  i_nominal_value=1  v_specify=off  v_priority=None  v=0 V  v_nominal_specify=off  v_nominal_unit=V  v_nominal_value=1
  Temperature Sensor : fl_lib/Thermal/Thermal Sensors/Temperature Sensor
  Thermal Mass : fl_lib/Thermal/Thermal Elements/Thermal Mass  mass=64 kg  sp_heat=346.875 J/(K*kg)  T_specify=on  T_priority=High  T=293.15 K  T_nominal_specify=off  T_nominal_unit=K  T_nominal_value=1  Q_specify=off  Q_priority=None  Q=0 W  Q_nominal_specify=off  Q_nominal_unit=W  Q_nominal_value=1
  Thermal Reference : fl_lib/Thermal/Thermal Elements/Thermal Reference
  Thermal Resistor{,1,3..8} (8 alike) : fl_lib/Electrical/Electrical Elements/Thermal Resistor  R0=208^2/1718*8 Ohm  T0=298.15 K  alpha=50e-6 1/K  tc=10 s  K_d=1e-3 W/K  T_specify=on  T_priority=High  T=293.15 K  T_nominal_specify=off  T_nominal_unit=K  T_nominal_value=1
      settings: SourceProductBaseCode=SS  InternalSimscapePortConfiguration="{\"Bottom\":[],\"Left\":[{\"id\":\"H\",\"label\":\"H\",\"type\":\"foundation.thermal.thermal\"},{\"id\":\"p\",\"label\":\"+\",\"type\":\"foundation.electrical.electrical\"}],\"Right\":[{\"id\":\"n\",\"label\":\"-\",\"type\":\"foundation.electrical.electrical\"}],\"Top\":[]}"
  Intake : PMIOPort  Side=Left
  Exhaust : PMIOPort  Port=2  Side=Right
  Out1 : Outport
  Out2 : Outport  Port=2
  Out3 : Outport  Port=3
  wires:
  Demux/6 -> Simulink-PS Converter5/1
  Demux/1 -> Simulink-PS Converter2/1
  Demux/2 -> Simulink-PS Converter1/1
  Demux/7 -> Simulink-PS Converter6/1
  PS-Simulink Converter2/1 -> Out1/1, [Temp]  "temperature"
  [Curr] -> Scope/2, Gain1/1  "current"
  [Temp] -> Scope/1  "temperature"
  PS-Simulink Converter3/1 -> [Curr]
  Saturation/1 -> MATLAB Function/1(load)
  In2/1 -> Saturation/1  "demand"
  Demux/4 -> Simulink-PS Converter3/1
  Demux/3 -> Simulink-PS Converter/1
  Demux/5 -> Simulink-PS Converter4/1
  MATLAB Function/1(s) -> Demux/1
  Gain1/1 -> Out2/1, Scope/3  "operational power"
  In1/1 -> Gain/1, Gain2/1  "fan"
  Gain2/1 -> Simulink-PS Converter7/1
  Gain/1 -> Out3/1  "cooling power"
  PS-Simulink Converter5/1 -> Scope2/1  "room pressure"
  PS-Simulink Converter4/1 -> Scope2/2  "room temperature"
  connections:
  Switch3/LConn1 -- Switch2/RConn2 -- Thermal Resistor3/LConn2
  Thermal Resistor3/RConn1 -- Thermal Resistor6/RConn1 -- Thermal Resistor7/RConn1 -- Thermal Resistor5/RConn1 -- Thermal Resistor4/RConn1 -- Thermal Resistor8/RConn1 -- Electrical Reference/LConn1 -- DC Voltage Source/RConn1 -- Thermal Resistor/RConn1 -- Thermal Resistor1/RConn1
  DC Voltage Source/LConn1 -- Current Sensor/LConn1
  Switch2/LConn1 -- Switch1/RConn2 -- Thermal Resistor1/LConn2
  Switch1/LConn1 -- Switch/RConn2 -- Thermal Resistor8/LConn2
  Thermal Resistor4/LConn2 -- Switch4/LConn1 -- Switch3/RConn2
  Switch6/LConn1 -- Switch5/RConn2 -- Thermal Resistor6/LConn2
  Switch/LConn1 -- Current Sensor/RConn2 -- Thermal Resistor/LConn2
  Thermal Resistor5/LConn2 -- Switch5/LConn1 -- Switch4/RConn2
  Thermal Reference/LConn1 -- Temperature Sensor/RConn1
  Simulink-PS Converter6/RConn1 -- Switch6/RConn1
  Thermal Resistor7/LConn2 -- Switch6/RConn2
  Simulink-PS Converter4/RConn1 -- Switch4/RConn1
  Simulink-PS Converter2/RConn1 -- Switch/RConn1
  Simulink-PS Converter1/RConn1 -- Switch1/RConn1
  Temperature Sensor/RConn2 -- PS-Simulink Converter2/LConn1
  Simulink-PS Converter/RConn1 -- Switch2/RConn1
  Current Sensor/RConn1 -- PS-Simulink Converter3/LConn1
  Simulink-PS Converter3/RConn1 -- Switch3/RConn1
  Simulink-PS Converter5/RConn1 -- Switch5/RConn1
  Controlled Volumetric Flow Rate Source (MA)/LConn2 -- Simulink-PS Converter7/RConn1
  Pipe (MA)/RConn1 -- Controlled Volumetric Flow Rate Source (MA)/RConn1 -- Pressure & Temperature Sensor (MA)1/LConn1
  Intake/RConn1 -- Controlled Volumetric Flow Rate Source (MA)/LConn1
  Pipe (MA)/LConn1 -- Exhaust/RConn1
  Thermal Resistor8/LConn1 -- Pipe (MA)/LConn2 -- Temperature Sensor/LConn1 -- Thermal Resistor/LConn1 -- Thermal Mass/LConn1 -- Thermal Resistor6/LConn1 -- Thermal Resistor7/LConn1 -- Thermal Resistor5/LConn1 -- Thermal Resistor4/LConn1 -- Thermal Resistor3/LConn1 -- Thermal Resistor1/LConn1
  PS-Simulink Converter5/LConn1 -- Pressure & Temperature Sensor (MA)1/RConn2
  PS-Simulink Converter4/LConn1 -- Pressure & Temperature Sensor (MA)1/RConn3
  Absolute Reference (MA)1/LConn1 -- Pressure & Temperature Sensor (MA)1/RConn1

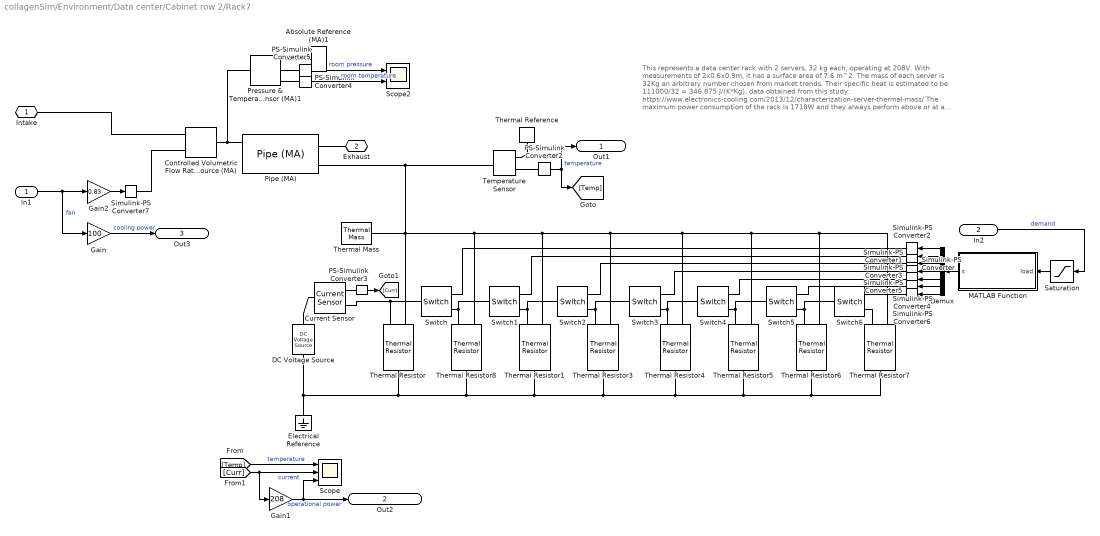
== system collagenSim/Environment/Data center/Cabinet row 2/Rack7 ==
  note: This represents a data center rack with 2 servers, 32 kg each, operating at 208V. With measurements of 2x0.6x0.9m, it has a surface area of 7.6 m^2. The mass of each server is 32Kg an arbitrary number chosen from market trends. Their specific heat is estimated to be 111000/32 = 346.875 J/(K*Kg), data obtained from this study: https://www.electronics-cooling.com/2013/12/characterization-server-thermal-mass/
      | The maximum power consumption of the rack is 1718W and they always perform above or at a minumum of 214.75W.
      | The rack's temperature exchange with the outside environment is modeled with a fluid pipe using the thermal propeties of air at sea level. The cooling system is modeled as eight 8mm four fan panels consuming a maximum of 100W per panel, which gives to each of the eight a total maximum vulumetric rate of 212m^3/min, meaning 0.83m^3/s. The surface area of the pipe representing the interior of the servers has been underestimated to be equal to the surface of the casing that contains them.
  In1 : Inport
  In2 : Inport  Port=2
  Absolute Reference (MA)1 : fl_lib/Moist Air/Elements/Absolute Reference (MA)
      settings: SourceProductBaseCode=SS
  Controlled Volumetric Flow Rate Source (MA) : fl_lib/Moist Air/Sources/Controlled Volumetric Flow Rate Source (MA)  power_spec=foundation.enum.power_spec.isentropic  volumetric_flow_conditions=foundation.enum.volumetric_flow_conditions.actual  p_std=0.101325 MPa  T_std=20 degC  RH_std=0.65  area_A=2*(2*0.442*0.4+2*0.442*0.711) m^2  area_B=2*(2*0.442*0.4+2*0.442*0.711) m^2
      settings: SourceProductBaseCode=SS  InternalSimscapePortConfiguration="{\"Bottom\":[],\"Left\":[{\"id\":\"A\",\"label\":\"A\",\"type\":\"foundation.moist_air.moist_air\"},{\"id\":\"V\",\"label\":\"V\",\"type\":\"input\"}],\"Right\":[{\"id\":\"B\",\"label\":\"B\",\"type\":\"foundation.moist_air.moist_air\"}],\"Top\":[]}"
  Current Sensor : fl_lib/Electrical/Electrical Sensors/Current Sensor
  DC Voltage Source : fl_lib/Electrical/Electrical Sources/DC Voltage Source  v0=208 V
  Demux : Demux  Outputs=7
  Electrical Reference : fl_lib/Electrical/Electrical Elements/Electrical Reference
  Gain : Gain  Gain=100
  Gain1 : Gain  Gain=208
  Gain2 : Gain  Gain=0.83
  MATLAB Function : MATLAB Function  TreatAsAtomicUnit=on
  PS-Simulink Converter{2..5} (4 alike) : nesl_utility/PS-Simulink Converter  PhysicalDomain=network_engine_domain  SubClassName=ps_output  LeftPortType=input  RightPortType=output  PseudoPeriodic=off  Frequencies=[]  Unit=inherit  AffineConversion=off
      settings: SourceProductBaseCode=PW,SS
  Pipe (MA) : fl_lib/Moist Air/Elements/Pipe (MA)  length=0.711 m  area=2*(2*0.442*0.4+2*0.442*0.711) m^2  Dh=0.1 m  length_add=0.1 m  roughness=15e-6 m  Re_lam=2000  Re_tur=4000  shape_factor=64  Nu_lam=3.66  RH_ws=1  time_constant=1e-3 s  moisture_trace_gas_source=foundation.enum.moisture_trace_gas_source.none  moisture_source_spec=foundation.enum.moisture_source_spec.vapor  moisture_mass_flow=0 kg/s  moisture_temperature_spec=foundation.enum.temperature_spec.atmospheric  moisture_temperature=293.15 K  trace_gas_mass_flow=0 kg/s  trace_gas_temperature_spec=foundation.enum.temperature_spec.atmospheric  trace_gas_temperature=293.15 K  p_I_specify=off  p_I_priority=High  p_I=0.101325 MPa  p_I_nominal_specify=off  p_I_nominal_unit=MPa  p_I_nominal_value=1  T_I_specify=off  T_I_priority=High  T_I=293.15 K  T_I_nominal_specify=off  T_I_nominal_unit=K  T_I_nominal_value=1  RH_I_specify=off  RH_I_priority=High  RH_I=0  RH_I_nominal_specify=off  RH_I_nominal_unit=1  RH_I_nominal_value=1  x_w_I_specify=off  x_w_I_priority=None  x_w_I=0  x_w_I_nominal_specify=off  x_w_I_nominal_unit=1  x_w_I_nominal_value=1  y_w_I_specify=off  y_w_I_priority=None  y_w_I=0  y_w_I_nominal_specify=off  y_w_I_nominal_unit=1  y_w_I_nominal_value=1  HR_I_specify=off  HR_I_priority=None  HR_I=0  HR_I_nominal_specify=off  HR_I_nominal_unit=1  HR_I_nominal_value=1  x_g_I_specify=off  x_g_I_priority=High  x_g_I=0  x_g_I_nominal_specify=off  x_g_I_nominal_unit=1  x_g_I_nominal_value=1  y_g_I_specify=off  y_g_I_priority=None  y_g_I=0  y_g_I_nominal_specify=off  y_g_I_nominal_unit=1  y_g_I_nominal_value=1
      settings: SourceProductBaseCode=SS
  Pressure & Temperature Sensor (MA)1 : fl_lib/Moist Air/Sensors/Pressure & Temperature Sensor (MA)
      settings: SourceProductBaseCode=SS  InternalSimscapePortConfiguration="{\"Bottom\":[],\"Left\":[{\"id\":\"A\",\"label\":\"A\",\"type\":\"foundation.moist_air.moist_air\"}],\"Right\":[{\"id\":\"B\",\"label\":\"B\",\"type\":\"foundation.moist_air.moist_air\"},{\"id\":\"P\",\"label\":\"P\",\"type\":\"output\"},{\"id\":\"T\",\"label\":\"T\",\"type\":\"output\"}],\"Top\":[]}"
  Saturation : Saturate  UpperLimit=0.99  LowerLimit=0.01
  Scope : Scope  NumInputPorts=3
  Scope2 : Scope  NumInputPorts=2
  Simulink-PS Converter{,1..7} (8 alike) : nesl_utility/Simulink-PS Converter  PhysicalDomain=network_engine_domain  SubClassName=ps_input  LeftPortType=input  RightPortType=output  PseudoPeriodic=off  Frequencies=[]  NoiseDistribution=none  NoiseParameters=[]  Unit=1  AffineConversion=off  FilteringAndDerivatives=provide  SimscapeFilterOrder=1  InputFilterTimeConstant=0.001  UdotUserProvided=0
      settings: SourceProductBaseCode=PW,SS
  Switch{,1..6} (7 alike) : fl_lib/Electrical/Electrical Elements/Switch  R_closed=0.01 Ohm  G_open=1e-8 1/Ohm  Threshold=0.5  i_specify=off  i_priority=None  i=0 A  i_nominal_specify=off  i_nominal_unit=A  i_nominal_value=1  v_specify=off  v_priority=None  v=0 V  v_nominal_specify=off  v_nominal_unit=V  v_nominal_value=1
  Temperature Sensor : fl_lib/Thermal/Thermal Sensors/Temperature Sensor
  Thermal Mass : fl_lib/Thermal/Thermal Elements/Thermal Mass  mass=64 kg  sp_heat=346.875 J/(K*kg)  T_specify=on  T_priority=High  T=293.15 K  T_nominal_specify=off  T_nominal_unit=K  T_nominal_value=1  Q_specify=off  Q_priority=None  Q=0 W  Q_nominal_specify=off  Q_nominal_unit=W  Q_nominal_value=1
  Thermal Reference : fl_lib/Thermal/Thermal Elements/Thermal Reference
  Thermal Resistor{,1,3..8} (8 alike) : fl_lib/Electrical/Electrical Elements/Thermal Resistor  R0=208^2/1718*8 Ohm  T0=298.15 K  alpha=50e-6 1/K  tc=10 s  K_d=1e-3 W/K  T_specify=on  T_priority=High  T=293.15 K  T_nominal_specify=off  T_nominal_unit=K  T_nominal_value=1
      settings: SourceProductBaseCode=SS  InternalSimscapePortConfiguration="{\"Bottom\":[],\"Left\":[{\"id\":\"H\",\"label\":\"H\",\"type\":\"foundation.thermal.thermal\"},{\"id\":\"p\",\"label\":\"+\",\"type\":\"foundation.electrical.electrical\"}],\"Right\":[{\"id\":\"n\",\"label\":\"-\",\"type\":\"foundation.electrical.electrical\"}],\"Top\":[]}"
  Intake : PMIOPort  Side=Left
  Exhaust : PMIOPort  Port=2  Side=Right
  Out1 : Outport
  Out2 : Outport  Port=2
  Out3 : Outport  Port=3
  wires:
  Demux/6 -> Simulink-PS Converter5/1
  Demux/1 -> Simulink-PS Converter2/1
  Demux/2 -> Simulink-PS Converter1/1
  Demux/7 -> Simulink-PS Converter6/1
  PS-Simulink Converter2/1 -> Out1/1, [Temp]  "temperature"
  [Curr] -> Scope/2, Gain1/1  "current"
  [Temp] -> Scope/1  "temperature"
  PS-Simulink Converter3/1 -> [Curr]
  Saturation/1 -> MATLAB Function/1(load)
  In2/1 -> Saturation/1  "demand"
  Demux/4 -> Simulink-PS Converter3/1
  Demux/3 -> Simulink-PS Converter/1
  Demux/5 -> Simulink-PS Converter4/1
  MATLAB Function/1(s) -> Demux/1
  Gain1/1 -> Out2/1, Scope/3  "operational power"
  In1/1 -> Gain/1, Gain2/1  "fan"
  Gain2/1 -> Simulink-PS Converter7/1
  Gain/1 -> Out3/1  "cooling power"
  PS-Simulink Converter5/1 -> Scope2/1  "room pressure"
  PS-Simulink Converter4/1 -> Scope2/2  "room temperature"
  connections:
  Switch3/LConn1 -- Switch2/RConn2 -- Thermal Resistor3/LConn2
  Thermal Resistor3/RConn1 -- Thermal Resistor6/RConn1 -- Thermal Resistor7/RConn1 -- Thermal Resistor5/RConn1 -- Thermal Resistor4/RConn1 -- Thermal Resistor8/RConn1 -- Electrical Reference/LConn1 -- DC Voltage Source/RConn1 -- Thermal Resistor/RConn1 -- Thermal Resistor1/RConn1
  DC Voltage Source/LConn1 -- Current Sensor/LConn1
  Switch2/LConn1 -- Switch1/RConn2 -- Thermal Resistor1/LConn2
  Switch1/LConn1 -- Switch/RConn2 -- Thermal Resistor8/LConn2
  Thermal Resistor4/LConn2 -- Switch4/LConn1 -- Switch3/RConn2
  Switch6/LConn1 -- Switch5/RConn2 -- Thermal Resistor6/LConn2
  Switch/LConn1 -- Current Sensor/RConn2 -- Thermal Resistor/LConn2
  Thermal Resistor5/LConn2 -- Switch5/LConn1 -- Switch4/RConn2
  Thermal Reference/LConn1 -- Temperature Sensor/RConn1
  Simulink-PS Converter6/RConn1 -- Switch6/RConn1
  Thermal Resistor7/LConn2 -- Switch6/RConn2
  Simulink-PS Converter4/RConn1 -- Switch4/RConn1
  Simulink-PS Converter2/RConn1 -- Switch/RConn1
  Simulink-PS Converter1/RConn1 -- Switch1/RConn1
  Temperature Sensor/RConn2 -- PS-Simulink Converter2/LConn1
  Simulink-PS Converter/RConn1 -- Switch2/RConn1
  Current Sensor/RConn1 -- PS-Simulink Converter3/LConn1
  Simulink-PS Converter3/RConn1 -- Switch3/RConn1
  Simulink-PS Converter5/RConn1 -- Switch5/RConn1
  Controlled Volumetric Flow Rate Source (MA)/LConn2 -- Simulink-PS Converter7/RConn1
  Pipe (MA)/RConn1 -- Controlled Volumetric Flow Rate Source (MA)/RConn1 -- Pressure & Temperature Sensor (MA)1/LConn1
  Intake/RConn1 -- Controlled Volumetric Flow Rate Source (MA)/LConn1
  Pipe (MA)/LConn1 -- Exhaust/RConn1
  Thermal Resistor8/LConn1 -- Pipe (MA)/LConn2 -- Temperature Sensor/LConn1 -- Thermal Resistor/LConn1 -- Thermal Mass/LConn1 -- Thermal Resistor6/LConn1 -- Thermal Resistor7/LConn1 -- Thermal Resistor5/LConn1 -- Thermal Resistor4/LConn1 -- Thermal Resistor3/LConn1 -- Thermal Resistor1/LConn1
  PS-Simulink Converter5/LConn1 -- Pressure & Temperature Sensor (MA)1/RConn2
  PS-Simulink Converter4/LConn1 -- Pressure & Temperature Sensor (MA)1/RConn3
  Absolute Reference (MA)1/LConn1 -- Pressure & Temperature Sensor (MA)1/RConn1
